simulink model "prob3_week3"  (R2020b)
settings: Solver=VariableStepAuto  StartTime=0.0  StopTime=10.0  RelTol=1e-3
undefined symbols (not defined in the file): g, J, m, R, Tbmax
settings Model: Creator=Pulkit Khandelwal  LastModifiedBy=Pulkit Khandelwal

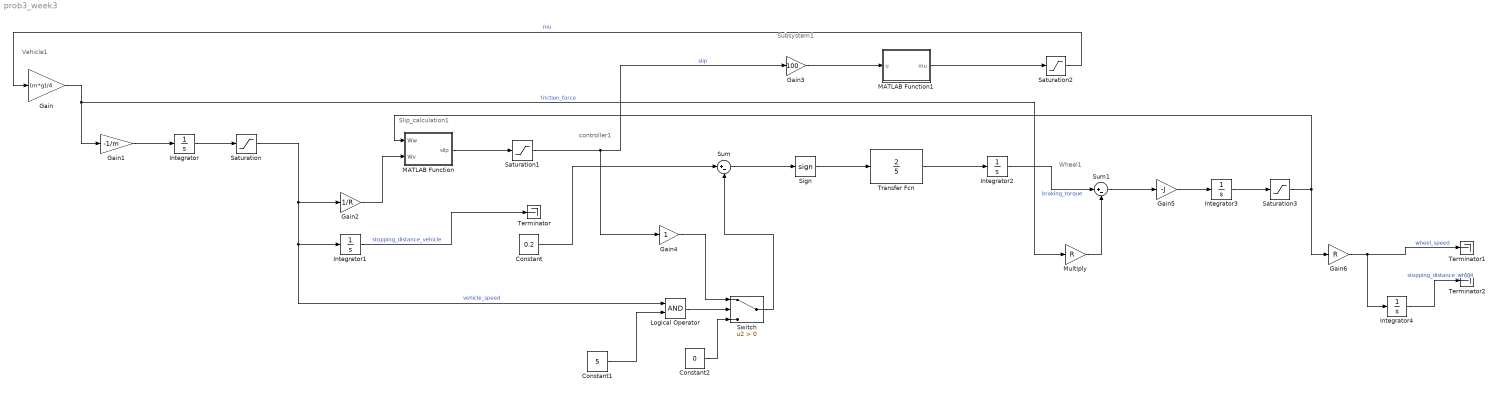
== system prob3_week3 ==
  note: Wheel1
  note: controller1
  note: Subsystem1
  note: Slip_calculation1
  note: Vehicle1
  Constant : Constant  Value=0.2
  Constant1 : Constant  Value=5  SampleTime=5
  Constant2 : Constant  Value=0
  Gain : Gain  Gain=(m*g)/4
  Gain1 : Gain  Gain=-1/m
  Gain2 : Gain  Gain=1/R
  Gain3 : Gain  Gain=100
  Gain4 : Gain
  Gain5 : Gain  Gain=-J
  Gain6 : Gain  Gain=R
  Integrator : Integrator  InitialCondition=2
  Integrator1 : Integrator
  Integrator2 : Integrator  LimitOutput=on  UpperSaturationLimit=Tbmax  LowerSaturationLimit=0
  Integrator3 : Integrator  InitialCondition=28/R
  Integrator4 : Integrator
  Logical Operator : Logic  AllPortsSameDT=off  OutDataTypeStr=boolean
  MATLAB Function : MATLAB Function  TreatAsAtomicUnit=on
  MATLAB Function1 : MATLAB Function  TreatAsAtomicUnit=on
  Multiply : Gain  Gain=R
  Saturation : Saturate  UpperLimit=1000  LowerLimit=0.001
  Saturation1 : Saturate  UpperLimit=1  LowerLimit=0
  Saturation2 : Saturate  UpperLimit=1  LowerLimit=0
  Saturation3 : Saturate  UpperLimit=1000  LowerLimit=0
  Sign : Signum
  Sum : Sum  Inputs=|+-
  Sum1 : Sum  Inputs=|+-
  Switch : Switch  Criteria=u2 > Threshold
  Terminator : Terminator
  Terminator1 : Terminator
  Terminator2 : Terminator
  Transfer Fcn : TransferFcn  Numerator=[2]  Denominator=5
  wires:
  Saturation1/1 -> Gain4/1, Gain3/1  "slip"
  Integrator1/1 -> Terminator/1  "stopping_distance_vehicle"
  Gain/1 -> Multiply/1, Gain1/1  "friction_force"
  Integrator4/1 -> Terminator2/1  "stopping_distance_wheel"
  Saturation/1 -> Logical Operator/1, Integrator1/1, Gain2/1  "vehicle_speed"
  Saturation2/1 -> Gain/1  "mu"
  Integrator2/1 -> Sum1/1  "braking_torque"
  Gain6/1 -> Terminator1/1, Integrator4/1  "wheel_speed"
  Integrator/1 -> Saturation/1
  Gain1/1 -> Integrator/1
  MATLAB Function/1(slip) -> Saturation1/1
  Gain2/1 -> MATLAB Function/2(Wv)
  Saturation3/1 -> MATLAB Function/1(Ww), Gain6/1
  MATLAB Function1/1(mu) -> Saturation2/1
  Gain3/1 -> MATLAB Function1/1(u)
  Transfer Fcn/1 -> Integrator2/1
  Sign/1 -> Transfer Fcn/1
  Sum/1 -> Sign/1
  Gain4/1 -> Switch/1
  Constant1/1 -> Logical Operator/2
  Constant2/1 -> Switch/3
  Switch/1 -> Sum/2
  Constant/1 -> Sum/1
  Logical Operator/1 -> Switch/2
  Integrator3/1 -> Saturation3/1
  Gain5/1 -> Integrator3/1
  Sum1/1 -> Gain5/1
  Multiply/1 -> Sum1/2

== matlab function prob3_week3/MATLAB Function1 ==
  data: u input; mu output
function mu = fcn(u)

mu=0.7*(1.07*(1-exp(-0.5*u)-0.003*u));

== matlab function prob3_week3/MATLAB Function ==
  data: Ww input; slip output; Wv input
function slip = fcn(Ww, Wv)

slip=1-(Ww/(Wv+(Wv==0)*eps));
